simulink model "Lithium0x2DionScaling"  (R2024b)
settings: Solver=FixedStepAuto  StartTime=0.0  StopTime=10  FixedStep=0.001  RelTol=1e-3
libraries: spsControlledCurrentSourceLib x1, spsControlledVoltageSourceLib x1, spsCurrentMeasurementLib x1, spsSeriesRLCBranchLib x1, spsVoltageMeasurementLib x1, spspowerguiLib x1
settings Model: Creator=holthoff  LastModifiedBy=kauchr

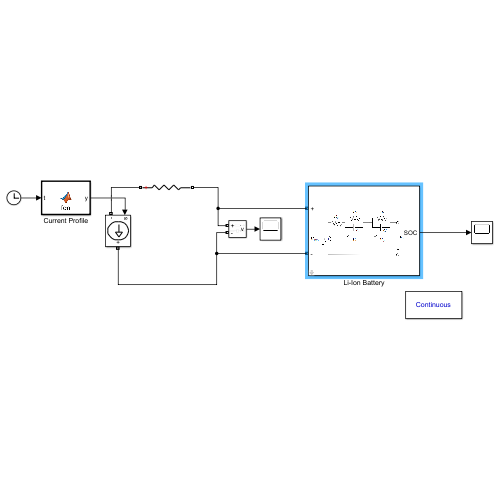
[thumbnail: Simulink's stored preview of the top-level diagram]
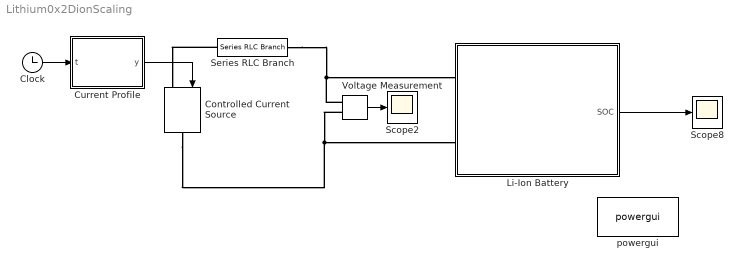
== system Lithium0x2DionScaling ==
  Clock : Clock
  Controlled Current Source : spsControlledCurrentSourceLib/Controlled Current Source  Initialize=off  Source_Type=AC  Amplitude=0  Phase=0  Frequency=0  Measurements=None
  Current Profile : MATLAB Function  TreatAsAtomicUnit=on
  Li-Ion Battery : Subsystem  mask{RCap=2.6, NomV=3.2, soc=50, n=100, m=100}
      mask prompts: RCap "Rated Capacity (Ah)"; NomV "Nominal Voltage (V)"; soc "Initial SOC (%)"; n "Number of cells in series"; m "Number of cells in parallel"
      mask DialogControl DescTextVar Prompt: Lithium-Ion Battery
      mask DialogControl Control2 Prompt: This generic model represents a lithium-ion battery consisting of an arbitrary number of cells connected in series and in parallel. The model is designed to simulate the electrical characteristics of the stack, including current, voltage, and SOC.
      mask Display: image('liion.png', [0,0,20,0,100,100]);
  Scope2 : Scope
  Scope8 : Scope
  Series RLC Branch : spsSeriesRLCBranchLib/Series RLC Branch  LConnTagsString=__new0  RConnTagsString=__new0  BranchType=R  Resistance=1  Inductance=1e-3  SetiL0=off  InitialCurrent=0  Capacitance=1e-6  Setx0=off  InitialVoltage=0  Measurements=None
  Voltage Measurement : spsVoltageMeasurementLib/Voltage Measurement  PhasorSimulation=off  OutputType=Complex  PSBequivalent=0
  powergui : spspowerguiLib/powergui  Priority=1  SimulationMode=Continuous  SampleTime=50e-6  frequency=60  Iterations=50  frequencyindice=0  Pbase=100e6  ErrMax=1e-4  UnitsV=kV  UnitsW=MW  buscounter=0  FunctionMessages=off  echomessages=off  EnableUseOfTLC=off  CurrentSourceSwitches=off  DisableSnubberDevices=off  DisableRonSwitches=off  DisableVfSwitches=off  DisplayEquations=off  AutomaticDiscreteSolvers=off  SolverType=Tustin/Backward Euler (TBE)  Interpol=off  ExternalGateDelay=off  methode=off  Ts=100  x0status=blocks  SPID=on  SwTol=0  HookPort=off  NonlinearTolerance=1e-4  nMaxIteration=100  ContinueOnMaxIteration=off  RestoreLinks=warning  ResistiveCurrentMeasurement=off  Frange=[0:2:500]  Ylog=off  Xlog=on  ShowGrid=off  save=off  variable=ZData  structure=0  ZoomFFT=off  StartTime=0.0  cycles=1  DisplayStyle=1  fundamental=60  FreqAxis=off  MaxFrequency=1000  frequencyindicesteady=1  RmsSteady=1  display=off
  wires:
  Li-Ion Battery/1(SOC) -> Scope8/1
  Clock/1 -> Current Profile/1(t)
  Voltage Measurement/1 -> Scope2/1
  Current Profile/1(y) -> Controlled Current Source/1
  connections:
  Controlled Current Source/RConn1 -- Voltage Measurement/LConn2 -- Li-Ion Battery/LConn2
  Voltage Measurement/LConn1 -- Series RLC Branch/RConn1 -- Li-Ion Battery/LConn1
  Series RLC Branch/LConn1 -- Controlled Current Source/LConn1

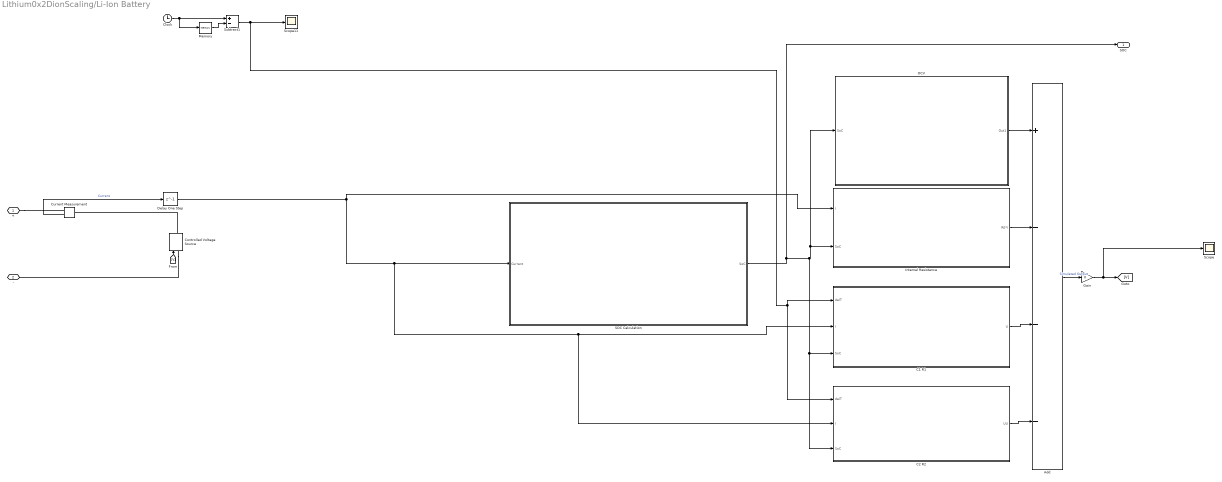
== system Lithium0x2DionScaling/Li-Ion Battery ==
  Add : Sum  Inputs=+---
  C1 R1 : Subsystem
  C2 R2 : Subsystem
  Clock : Clock
  Controlled Voltage Source : spsControlledVoltageSourceLib/Controlled Voltage Source  Initialize=on  Source_Type=AC  Amplitude=0  Phase=0  Frequency=0  Measurements=None
  Current Measurement : spsCurrentMeasurementLib/Current Measurement  PhasorSimulation=off  OutputType=Complex  PSBequivalent=0
  Delay One Step : Delay  DelayLength=1
  Gain : Gain  Gain=n
  Internal Resistance : Subsystem
  Memory : Memory
  OCV : Subsystem
  SOC Calculation : Subsystem
  Scope : Scope
  Scope11 : Scope
  Subtract1 : Sum  Inputs=+-
  + : PMIOPort  Side=Left
  - : PMIOPort  Port=2  Side=Left
  SOC : Outport
  wires:
  Add/1 -> Gain/1  "Simulated Output"
  Clock/1 -> Subtract1/1, Memory/1
  Subtract1/1 -> C2 R2/1(delT), C1 R1/1(delT), Scope11/1
  Memory/1 -> Subtract1/2
  Internal Resistance/1(R0*I) -> Add/2
  OCV/1(Out1) -> Add/1
  C1 R1/1(U) -> Add/3
  C2 R2/1(UU) -> Add/4
  SOC Calculation/1(SoC) -> SOC/1, OCV/1(SoC), Internal Resistance/2(SoC), C2 R2/3(SoC), C1 R1/3(SoC)
  [V] -> Controlled Voltage Source/1
  Current Measurement/1 -> Delay One Step/1  "Current"
  Delay One Step/1 -> C2 R2/2(I), C1 R1/2(I), SOC Calculation/1(Current), Internal Resistance/1(I)
  Gain/1 -> Scope/1, [V]
  connections:
  +/RConn1 -- Current Measurement/RConn1
  Controlled Voltage Source/RConn1 -- Current Measurement/LConn1
  Controlled Voltage Source/LConn1 -- -/RConn1

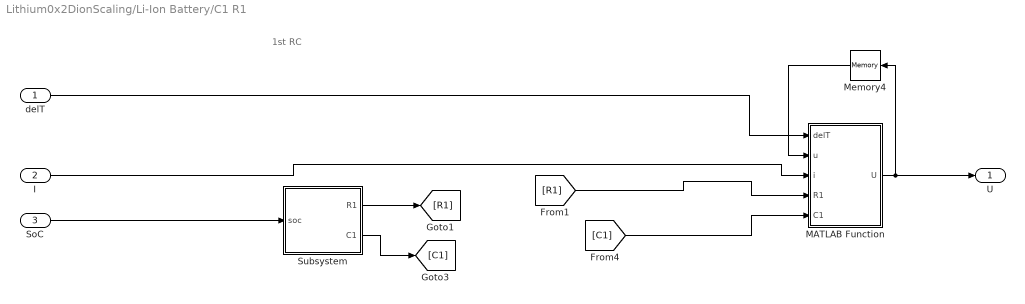
== system Lithium0x2DionScaling/Li-Ion Battery/C1 R1 ==
  note: 1st RC
  delT : Inport
  I : Inport  Port=2
  SoC : Inport  Port=3
  MATLAB Function : MATLAB Function  TreatAsAtomicUnit=on
  Memory4 : Memory
  Subsystem : Subsystem
  U : Outport
  wires:
  Subsystem/1(R1) -> [R1]
  MATLAB Function/1(U) -> U/1, Memory4/1
  delT/1 -> MATLAB Function/1(delT)
  Memory4/1 -> MATLAB Function/2(u)
  [R1] -> MATLAB Function/4(R1)
  Subsystem/2(C1) -> [C1]
  [C1] -> MATLAB Function/5(C1)
  SoC/1 -> Subsystem/1(soc)
  I/1 -> MATLAB Function/3(i)

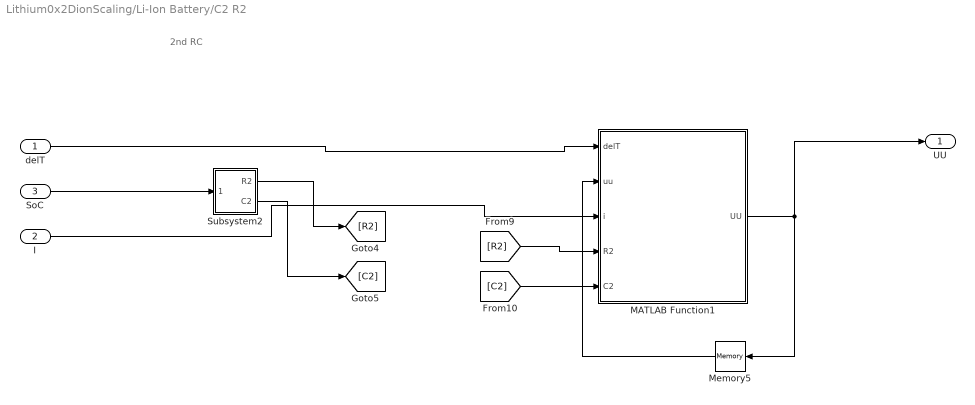
== system Lithium0x2DionScaling/Li-Ion Battery/C2 R2 ==
  note: 2nd RC
  delT : Inport
  I : Inport  Port=2
  SoC : Inport  Port=3
  MATLAB Function1 : MATLAB Function  TreatAsAtomicUnit=on
  Memory5 : Memory
  Subsystem2 : Subsystem
  UU : Outport
  wires:
  [R2] -> MATLAB Function1/4(R2)
  Subsystem2/2(C2) -> [C2]
  Memory5/1 -> MATLAB Function1/2(uu)
  Subsystem2/1(R2) -> [R2]
  [C2] -> MATLAB Function1/5(C2)
  MATLAB Function1/1(UU) -> UU/1, Memory5/1
  SoC/1 -> Subsystem2/1(soc)
  delT/1 -> MATLAB Function1/1(delT)
  I/1 -> MATLAB Function1/3(i)

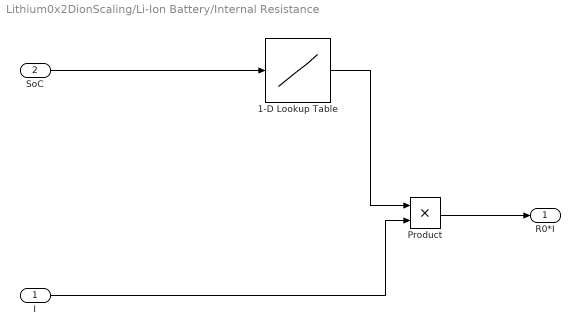
== system Lithium0x2DionScaling/Li-Ion Battery/Internal Resistance ==
  I : Inport
  SoC : Inport  Port=2
  1-D Lookup Table : Lookup_n-D  NumberOfTableDimensions=1  BreakpointsForDimension1=[0;0.01;0.02;0.029999999999999999;0.040000000000000001;0.050000000000000003;0.059999999999999998;0.070000000000000007;0.080000000000000002;0.089999999999999997;0.10000000000000001;0.11;0.12;0.13;0.14000000000000001;0.14999999999999999;0.16;0.17000000000000001;0.17999999999999999;0.19;0.20000000000000001;0.20999999999999999;0.22;0.23000000000000001;0.23999999999999999;0.25;0.26000000000000001;0.27000000000000002;0.28000000000000003;0.28999999999999998;0.29999999999999999;0.31;0.32000000000000001;0.33000000000000002;0.34000000000000002;0.34999999999999998;0.35999999999999999;0.37;0.38;0.39000000000000001;0.40000000000000002;0.40999999999999998;0.41999999999999998;0.42999999999999999;0.44;0.45000000000000001;0.46000000000000002;0.46999999999999997;0.47999999999999998;0.48999999999999999;0.5;0.51000000000000001;0.52000000000000002;0.53000000000000003;0.54000000000000004;0.55000000000000004;0.56000000000000005;0.56999999999999995;0.57999999999999996;0.58999999999999997;0.59999999999999998;0.60999999999999999;0.62;0.63;0.64000000000000001;0.65000000000000002;0.66000000000000003;0.67000000000000004;0.68000000000000005;0.68999999999999995;0.69999999999999996;0.70999999999999996;0.71999999999999997;0.72999999999999998;0.73999999999999999;0.75;0.76000000000000001;0.77000000000000002;0.78000000000000003;0.79000000000000004;0.80000000000000004;0.81000000000000005;0.81999999999999995;0.82999999999999996;0.83999999999999997;0.84999999999999998;0.85999999999999999;0.87;0.88;0.89000000000000001;0.90000000000000002;0.91000000000000003;0.92000000000000004;0.93000000000000005;0.93999999999999995;0.94999999999999996;0.95999999999999996;0.96999999999999997;0.97999999999999998;0.98999999999999999;1]  Table=[0.0263338;0.01843229;0.01552549;0.01445614;0.01406275;0.01391803;0.01386479;0.0138452;0.01383799;0.01383534;0.01383437;0.01383401;0.01383388;0.01383383;0.01383381;0.01383381;0.0138338;0.0138338;0.0138338;0.0138338;0.0138338;0.0138338;0.0138338;0.0138338;0.0138338;0.0138338;0.0138338;0.0138338;0.0138338;0.0138338;0.0138338;0.0138338;0.0138338;0.0138338;0.0138338;0.0138338;0.0138338;0.0138338;0.0138338;0.0138338;0.0138338;0.0138338;0.0138338;0.0138338;0.0138338;0.0138338;0.0138338;0.0138338;0.0138338;0.0138338;0.0138338;0.0138338;0.0138338;0.0138338;0.0138338;0.0138338;0.0138338;0.0138338;0.0138338;0.0138338;0.0138338;0.0138338;0.0138338;0.0138338;0.0138338;0.0138338;0.0138338;0.0138338;0.0138338;0.0138338;0.0138338;0.0138338;0.0138338;0.0138338;0.0138338;0.0138338;0.0138338;0.0138338;0.0138338;0.0138338;0.0138338;0.0138338;0.0138338;0.0138338;0.0138338;0.0138338;0.0138338;0.0138338;0.0138338;0.0138338;0.0138338;0.0138338;0.0138338;0.0138338;0.0138338;0.0138338;0.0138338;0.0138338;0.0138338;0.0138338;0.0138338]  InternalRulePriority=Speed  RndMeth=Simplest
  Product : Product
  R0*I : Outport
  wires:
  Product/1 -> R0*I/1
  SoC/1 -> 1-D Lookup Table/1
  I/1 -> Product/2
  1-D Lookup Table/1 -> Product/1

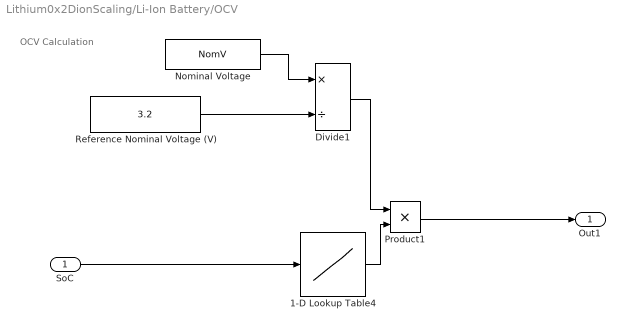
== system Lithium0x2DionScaling/Li-Ion Battery/OCV ==
  note: OCV Calculation
  SoC : Inport
  1-D Lookup Table4 : Lookup_n-D  NumberOfTableDimensions=1  BreakpointsForDimension1=[0;0.01;0.02;0.029999999999999999;0.040000000000000001;0.050000000000000003;0.059999999999999998;0.070000000000000007;0.080000000000000002;0.089999999999999997;0.10000000000000001;0.11;0.12;0.13;0.14000000000000001;0.14999999999999999;0.16;0.17000000000000001;0.17999999999999999;0.19;0.20000000000000001;0.20999999999999999;0.22;0.23000000000000001;0.23999999999999999;0.25;0.26000000000000001;0.27000000000000002;0.28000000000000003;0.28999999999999998;0.29999999999999999;0.31;0.32000000000000001;0.33000000000000002;0.34000000000000002;0.34999999999999998;0.35999999999999999;0.37;0.38;0.39000000000000001;0.40000000000000002;0.40999999999999998;0.41999999999999998;0.42999999999999999;0.44;0.45000000000000001;0.46000000000000002;0.46999999999999997;0.47999999999999998;0.48999999999999999;0.5;0.51000000000000001;0.52000000000000002;0.53000000000000003;0.54000000000000004;0.55000000000000004;0.56000000000000005;0.56999999999999995;0.57999999999999996;0.58999999999999997;0.59999999999999998;0.60999999999999999;0.62;0.63;0.64000000000000001;0.65000000000000002;0.66000000000000003;0.67000000000000004;0.68000000000000005;0.68999999999999995;0.69999999999999996;0.70999999999999996;0.71999999999999997;0.72999999999999998;0.73999999999999999;0.75;0.76000000000000001;0.77000000000000002;0.78000000000000003;0.79000000000000004;0.80000000000000004;0.81000000000000005;0.81999999999999995;0.82999999999999996;0.83999999999999997;0.84999999999999998;0.85999999999999999;0.87;0.88;0.89000000000000001;0.90000000000000002;0.91000000000000003;0.92000000000000004;0.93000000000000005;0.93999999999999995;0.94999999999999996;0.95999999999999996;0.96999999999999997;0.97999999999999998;0.98999999999999999;1]  Table=[3.29571729606682;3.32213631956766;3.34664360147367;3.36934563044947;3.39034548891849;3.40974290407478;3.42763429889471;3.44411284314879;3.45926850441342;3.47318809908262;3.48595534337984;3.49765090436971;3.50835245096978;3.51813470496231;3.52706949200605;3.53522579264794;3.54266979333496;3.54946493742581;3.55567197620274;3.56134901988328;3.56655158863201;3.57133266357232;3.5757427377982;3.57982986738595;3.58363972240603;3.58721563793471;3.59059866506595;3.59382762192308;3.59693914467061;3.59996773852596;3.60294582877126;3.60590381176509;3.60887010595426;3.61187120288554;3.61493171821749;3.61807444273214;3.62132039334682;3.62468886412591;3.62819747729257;3.63186223424055;3.63569756654593;3.63971638697887;3.64393014051541;3.64834885534923;3.65298119390336;3.65783450384201;3.66291486908231;3.66822716080606;3.67377508847152;3.67956125082515;3.68558718691339;3.69185342709441;3.69835954404988;3.70510420379676;3.71208521669903;3.71929958847944;3.72674357123133;3.73441271443036;3.74230191594627;3.75040547305464;3.75871713344867;3.76723014625097;3.77593731302525;3.78483103878816;3.793903383021;3.80314611068152;3.81255074321565;3.82210860956932;3.83181089720015;3.84164870308928;3.85161308475308;3.86169511125496;3.87188591421712;3.88217673883228;3.8925589948755;3.90302430771591;3.91356456932847;3.92417198930575;3.9348391458697;3.94555903688339;3.95632513086279;3.96713141798853;3.97797246111767;3.98884344679546;3.99974023626709;4.01065941648949;4.02159835114304;4.03255523164341;4.04352912815324;4.05452004059395;4.06552894965752;4.07655786781822;4.08760989034436;4.09868924631014;4.10980134960729;4.12095284995694;4.13215168392133;4.14340712591558;4.15472983921947;4.16613192698919;4.17762698326911]  InternalRulePriority=Speed  RndMeth=Simplest
  Divide1 : Product  Inputs=*/
  Nominal Voltage : Constant  Value=NomV
  Product1 : Product
  Reference Nominal Voltage (V) : Constant  Value=3.2
  Out1 : Outport
  wires:
  Product1/1 -> Out1/1
  1-D Lookup Table4/1 -> Product1/2
  SoC/1 -> 1-D Lookup Table4/1
  Reference Nominal Voltage (V)/1 -> Divide1/2
  Divide1/1 -> Product1/1
  Nominal Voltage/1 -> Divide1/1

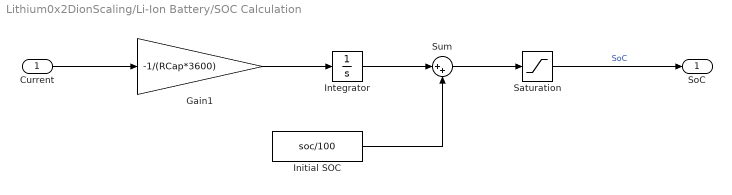
== system Lithium0x2DionScaling/Li-Ion Battery/SOC Calculation ==
  Current : Inport
  Gain1 : Gain  Gain=-1/(RCap*3600)
  Initial SOC : Constant  Value=soc/100
  Integrator : Integrator
  Saturation : Saturate  UpperLimit=1  LowerLimit=0
  Sum : Sum  Inputs=|++
  SoC : Outport
  wires:
  Current/1 -> Gain1/1
  Gain1/1 -> Integrator/1
  Integrator/1 -> Sum/1
  Initial SOC/1 -> Sum/2
  Sum/1 -> Saturation/1
  Saturation/1 -> SoC/1  "SoC"

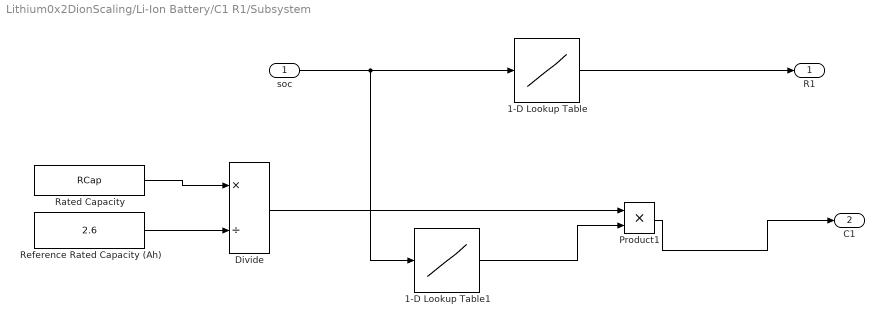
== system Lithium0x2DionScaling/Li-Ion Battery/C1 R1/Subsystem ==
  soc : Inport
  " Rated Capacity" : Constant  Value=RCap
  1-D Lookup Table : Lookup_n-D  NumberOfTableDimensions=1  BreakpointsForDimension1=[0;0.01;0.02;0.029999999999999999;0.040000000000000001;0.050000000000000003;0.059999999999999998;0.070000000000000007;0.080000000000000002;0.089999999999999997;0.10000000000000001;0.11;0.12;0.13;0.14000000000000001;0.14999999999999999;0.16;0.17000000000000001;0.17999999999999999;0.19;0.20000000000000001;0.20999999999999999;0.22;0.23000000000000001;0.23999999999999999;0.25;0.26000000000000001;0.27000000000000002;0.28000000000000003;0.28999999999999998;0.29999999999999999;0.31;0.32000000000000001;0.33000000000000002;0.34000000000000002;0.34999999999999998;0.35999999999999999;0.37;0.38;0.39000000000000001;0.40000000000000002;0.40999999999999998;0.41999999999999998;0.42999999999999999;0.44;0.45000000000000001;0.46000000000000002;0.46999999999999997;0.47999999999999998;0.48999999999999999;0.5;0.51000000000000001;0.52000000000000002;0.53000000000000003;0.54000000000000004;0.55000000000000004;0.56000000000000005;0.56999999999999995;0.57999999999999996;0.58999999999999997;0.59999999999999998;0.60999999999999999;0.62;0.63;0.64000000000000001;0.65000000000000002;0.66000000000000003;0.67000000000000004;0.68000000000000005;0.68999999999999995;0.69999999999999996;0.70999999999999996;0.71999999999999997;0.72999999999999998;0.73999999999999999;0.75;0.76000000000000001;0.77000000000000002;0.78000000000000003;0.79000000000000004;0.80000000000000004;0.81000000000000005;0.81999999999999995;0.82999999999999996;0.83999999999999997;0.84999999999999998;0.85999999999999999;0.87;0.88;0.89000000000000001;0.90000000000000002;0.91000000000000003;0.92000000000000004;0.93000000000000005;0.93999999999999995;0.94999999999999996;0.95999999999999996;0.96999999999999997;0.97999999999999998;0.98999999999999999;1]  Table=[0.025;0.01709849;0.01419169;0.01312234;0.01272895;0.01258422;0.01253098;0.0125114;0.01250419;0.01250154;0.01250057;0.01250021;0.01250008;0.01250003;0.01250001;0.0125;0.0125;0.0125;0.0125;0.0125;0.0125;0.0125;0.0125;0.0125;0.0125;0.0125;0.0125;0.0125;0.0125;0.0125;0.0125;0.0125;0.0125;0.0125;0.0125;0.0125;0.0125;0.0125;0.0125;0.0125;0.0125;0.0125;0.0125;0.0125;0.0125;0.0125;0.0125;0.0125;0.0125;0.0125;0.0125;0.0125;0.0125;0.0125;0.0125;0.0125;0.0125;0.0125;0.0125;0.0125;0.0125;0.0125;0.0125;0.0125;0.0125;0.0125;0.0125;0.0125;0.0125;0.0125;0.0125;0.0125;0.0125;0.0125;0.0125;0.0125;0.0125;0.0125;0.0125;0.0125;0.0125;0.0125;0.0125;0.0125;0.0125;0.0125;0.0125;0.0125;0.0125;0.0125;0.0125;0.0125;0.0125;0.0125;0.0125;0.0125;0.0125;0.0125;0.0125;0.0125;0.0125]  InternalRulePriority=Speed  RndMeth=Simplest
  1-D Lookup Table1 : Lookup_n-D  NumberOfTableDimensions=1  BreakpointsForDimension1=[0;0.01;0.02;0.029999999999999999;0.040000000000000001;0.050000000000000003;0.059999999999999998;0.070000000000000007;0.080000000000000002;0.089999999999999997;0.10000000000000001;0.11;0.12;0.13;0.14000000000000001;0.14999999999999999;0.16;0.17000000000000001;0.17999999999999999;0.19;0.20000000000000001;0.20999999999999999;0.22;0.23000000000000001;0.23999999999999999;0.25;0.26000000000000001;0.27000000000000002;0.28000000000000003;0.28999999999999998;0.29999999999999999;0.31;0.32000000000000001;0.33000000000000002;0.34000000000000002;0.34999999999999998;0.35999999999999999;0.37;0.38;0.39000000000000001;0.40000000000000002;0.40999999999999998;0.41999999999999998;0.42999999999999999;0.44;0.45000000000000001;0.46000000000000002;0.46999999999999997;0.47999999999999998;0.48999999999999999;0.5;0.51000000000000001;0.52000000000000002;0.53000000000000003;0.54000000000000004;0.55000000000000004;0.56000000000000005;0.56999999999999995;0.57999999999999996;0.58999999999999997;0.59999999999999998;0.60999999999999999;0.62;0.63;0.64000000000000001;0.65000000000000002;0.66000000000000003;0.67000000000000004;0.68000000000000005;0.68999999999999995;0.69999999999999996;0.70999999999999996;0.71999999999999997;0.72999999999999998;0.73999999999999999;0.75;0.76000000000000001;0.77000000000000002;0.78000000000000003;0.79000000000000004;0.80000000000000004;0.81000000000000005;0.81999999999999995;0.82999999999999996;0.83999999999999997;0.84999999999999998;0.85999999999999999;0.87;0.88;0.89000000000000001;0.90000000000000002;0.91000000000000003;0.92000000000000004;0.93000000000000005;0.93999999999999995;0.94999999999999996;0.95999999999999996;0.96999999999999997;0.97999999999999998;0.98999999999999999;1]  Table=[49;49.3934693402873;49.6321205588285;49.7768698398515;49.8646647167634;49.9179150013761;49.9502129316321;49.9698026165777;49.9816843611112;49.9888910034617;49.9932620530009;49.9959132285615;49.9975212478233;49.998496560807;49.9990881180344;49.9994469156298;49.9996645373721;49.999796531631;49.9998765901959;49.9999251481701;49.9999546000702;49.9999724635506;49.9999832982992;49.9999898699064;49.9999938557876;49.9999962733468;49.9999977396706;49.9999986290409;49.9999991684713;49.9999994956523;49.9999996940977;49.9999998144608;49.9999998874648;49.9999999317439;49.9999999586006;49.99999997489;49.99999998477;49.9999999907625;49.9999999943972;49.9999999966017;49.9999999979388;49.9999999987498;49.9999999992417;49.9999999995401;49.999999999721;49.9999999998308;49.9999999998974;49.9999999999377;49.9999999999622;49.9999999999771;49.9999999999861;49.9999999999916;49.9999999999949;49.9999999999969;49.9999999999981;49.9999999999988;49.9999999999993;49.9999999999996;49.9999999999997;49.9999999999998;49.9999999999999;49.9999999999999;49.9999999999999;50;50;50;50;50;50;50;50;50;50;50;50;50;50;50;50;50;50;50;50;50;50;50;50;50;50;50;50;50;50;50;50;50;50;50;50;50;50]  InternalRulePriority=Speed  RndMeth=Simplest
  Divide : Product  Inputs=*/
  Product1 : Product
  Reference Rated Capacity (Ah) : Constant  Value=2.6
  R1 : Outport
  C1 : Outport  Port=2
  wires:
  soc/1 -> 1-D Lookup Table1/1, 1-D Lookup Table/1
  1-D Lookup Table1/1 -> Product1/2
  Reference Rated Capacity (Ah)/1 -> Divide/2
  Divide/1 -> Product1/1
  " Rated Capacity"/1 -> Divide/1
  Product1/1 -> C1/1
  1-D Lookup Table/1 -> R1/1

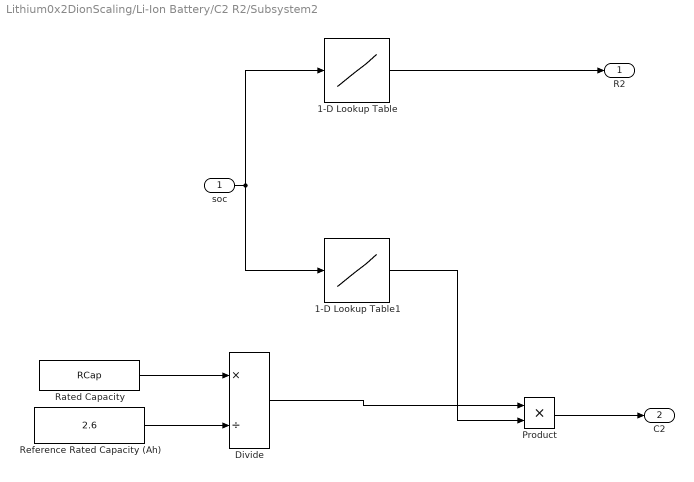
== system Lithium0x2DionScaling/Li-Ion Battery/C2 R2/Subsystem2 ==
  soc : Inport
  " Rated Capacity" : Constant  Value=RCap
  1-D Lookup Table : Lookup_n-D  NumberOfTableDimensions=1  BreakpointsForDimension1=[0;0.01;0.02;0.029999999999999999;0.040000000000000001;0.050000000000000003;0.059999999999999998;0.070000000000000007;0.080000000000000002;0.089999999999999997;0.10000000000000001;0.11;0.12;0.13;0.14000000000000001;0.14999999999999999;0.16;0.17000000000000001;0.17999999999999999;0.19;0.20000000000000001;0.20999999999999999;0.22;0.23000000000000001;0.23999999999999999;0.25;0.26000000000000001;0.27000000000000002;0.28000000000000003;0.28999999999999998;0.29999999999999999;0.31;0.32000000000000001;0.33000000000000002;0.34000000000000002;0.34999999999999998;0.35999999999999999;0.37;0.38;0.39000000000000001;0.40000000000000002;0.40999999999999998;0.41999999999999998;0.42999999999999999;0.44;0.45000000000000001;0.46000000000000002;0.46999999999999997;0.47999999999999998;0.48999999999999999;0.5;0.51000000000000001;0.52000000000000002;0.53000000000000003;0.54000000000000004;0.55000000000000004;0.56000000000000005;0.56999999999999995;0.57999999999999996;0.58999999999999997;0.59999999999999998;0.60999999999999999;0.62;0.63;0.64000000000000001;0.65000000000000002;0.66000000000000003;0.67000000000000004;0.68000000000000005;0.68999999999999995;0.69999999999999996;0.70999999999999996;0.71999999999999997;0.72999999999999998;0.73999999999999999;0.75;0.76000000000000001;0.77000000000000002;0.78000000000000003;0.79000000000000004;0.80000000000000004;0.81000000000000005;0.81999999999999995;0.82999999999999996;0.83999999999999997;0.84999999999999998;0.85999999999999999;0.87;0.88;0.89000000000000001;0.90000000000000002;0.91000000000000003;0.92000000000000004;0.93000000000000005;0.93999999999999995;0.94999999999999996;0.95999999999999996;0.96999999999999997;0.97999999999999998;0.98999999999999999;1]  Table=[0.025;0.01419169;0.01272895;0.01253098;0.01250419;0.01250057;0.01250008;0.01250001;0.0125;0.0125;0.0125;0.0125;0.0125;0.0125;0.0125;0.0125;0.0125;0.0125;0.0125;0.0125;0.0125;0.0125;0.0125;0.0125;0.0125;0.0125;0.0125;0.0125;0.0125;0.0125;0.0125;0.0125;0.0125;0.0125;0.0125;0.0125;0.0125;0.0125;0.0125;0.0125;0.0125;0.0125;0.0125;0.0125;0.0125;0.0125;0.0125;0.0125;0.0125;0.0125;0.0125;0.0125;0.0125;0.0125;0.0125;0.0125;0.0125;0.0125;0.0125;0.0125;0.0125;0.0125;0.0125;0.0125;0.0125;0.0125;0.0125;0.0125;0.0125;0.0125;0.0125;0.0125;0.0125;0.0125;0.0125;0.0125;0.0125;0.0125;0.0125;0.0125;0.0125;0.0125;0.0125;0.0125;0.0125;0.0125;0.0125;0.0125;0.0125;0.0125;0.0125;0.0125;0.0125;0.0125;0.0125;0.0125;0.0125;0.0125;0.0125;0.0125;0.0125]  InternalRulePriority=Speed  RndMeth=Simplest
  1-D Lookup Table1 : Lookup_n-D  NumberOfTableDimensions=1  BreakpointsForDimension1=[0;0.01;0.02;0.029999999999999999;0.040000000000000001;0.050000000000000003;0.059999999999999998;0.070000000000000007;0.080000000000000002;0.089999999999999997;0.10000000000000001;0.11;0.12;0.13;0.14000000000000001;0.14999999999999999;0.16;0.17000000000000001;0.17999999999999999;0.19;0.20000000000000001;0.20999999999999999;0.22;0.23000000000000001;0.23999999999999999;0.25;0.26000000000000001;0.27000000000000002;0.28000000000000003;0.28999999999999998;0.29999999999999999;0.31;0.32000000000000001;0.33000000000000002;0.34000000000000002;0.34999999999999998;0.35999999999999999;0.37;0.38;0.39000000000000001;0.40000000000000002;0.40999999999999998;0.41999999999999998;0.42999999999999999;0.44;0.45000000000000001;0.46000000000000002;0.46999999999999997;0.47999999999999998;0.48999999999999999;0.5;0.51000000000000001;0.52000000000000002;0.53000000000000003;0.54000000000000004;0.55000000000000004;0.56000000000000005;0.56999999999999995;0.57999999999999996;0.58999999999999997;0.59999999999999998;0.60999999999999999;0.62;0.63;0.64000000000000001;0.65000000000000002;0.66000000000000003;0.67000000000000004;0.68000000000000005;0.68999999999999995;0.69999999999999996;0.70999999999999996;0.71999999999999997;0.72999999999999998;0.73999999999999999;0.75;0.76000000000000001;0.77000000000000002;0.78000000000000003;0.79000000000000004;0.80000000000000004;0.81000000000000005;0.81999999999999995;0.82999999999999996;0.83999999999999997;0.84999999999999998;0.85999999999999999;0.87;0.88;0.89000000000000001;0.90000000000000002;0.91000000000000003;0.92000000000000004;0.93000000000000005;0.93999999999999995;0.94999999999999996;0.95999999999999996;0.96999999999999997;0.97999999999999998;0.98999999999999999;1]  Table=[299;299.632120558828;299.864664716763;299.950212931632;299.981684361111;299.993262053001;299.997521247823;299.999088118034;299.999664537372;299.999876590196;299.99995460007;299.999983298299;299.999993855787;299.99999773967;299.999999168471;299.999999694097;299.999999887464;299.9999999586;299.99999998477;299.999999994397;299.999999997939;299.999999999241;299.999999999721;299.999999999897;299.999999999962;299.999999999986;299.999999999995;299.999999999998;299.999999999999;299.999999999999;300;300;300;300;300;300;300;300;300;300;300;300;300;300;300;300;300;300;300;300;300;300;300;300;300;300;300;300;300;300;300;300;300;300;300;300;300;300;300;300;300;300;300;300;300;300;300;300;300;300;300;300;300;300;300;300;300;300;300;300;300;300;300;300;300;300;300;300;300;300;300]  InternalRulePriority=Speed  RndMeth=Simplest
  Divide : Product  Inputs=*/
  Product : Product
  Reference Rated Capacity (Ah) : Constant  Value=2.6
  R2 : Outport
  C2 : Outport  Port=2
  wires:
  1-D Lookup Table1/1 -> Product/2
  soc/1 -> 1-D Lookup Table1/1, 1-D Lookup Table/1
  Divide/1 -> Product/1
  Reference Rated Capacity (Ah)/1 -> Divide/2
  " Rated Capacity"/1 -> Divide/1
  Product/1 -> C2/1
  1-D Lookup Table/1 -> R2/1

== matlab function Lithium0x2DionScaling/Li-Ion Battery/C1 R1/MATLAB Function ==
  data: delT input; U output; u input; i input; R1 input; C1 input
function U    = fcn(delT,u, i, R1,C1)


 U = (exp(-delT/(R1*C1))*u)+(R1*(1-exp(-delT/(R1*C1)))*i);

== matlab function Lithium0x2DionScaling/Li-Ion Battery/C2 R2/MATLAB Function1 ==
  data: delT input; UU output; uu input; i input; R2 input; C2 input
function UU    = fcn(delT,uu, i, R2,C2)


 UU = (exp(-delT/(R2*C2))*uu)+(R2*(1-exp(-delT/(R2*C2)))*i);

== matlab function Lithium0x2DionScaling/Current Profile ==
  data: t input; y output
function y = fcn(t)
    ts = 0.001; % s
    t0 = 0;     % s
    tend = 5;   % s

    if t < t0 || t > tend
        y = 0; 
        return;
    end

    ms1 = 1.99; % s
    ms2 = 2;
    ms3 = 3;
    ms4 = 3.01;

    interval1 = t >= t0 && t < ms1;
    interval2 = t >= ms1 && t < ms2;
    interval3 = t >= ms2 && t < ms3;
    interval4 = t >= ms3 && t < ms4;
    interval5 = t >= ms4 && t <= tend;

    fvseg1 = 0;     % Final value of interval
    fvseg2 = 30;  % Rated maximum current peak current for 1 s in A
    fvseg3 = 30;
    fvseg4 = -32.5;
    fvseg5 = -32.5;

    if interval1
        y = fvseg1; 
    elseif interval2
        % Ramp up
        y = fvseg1 + (fvseg2 - fvseg1) * ((t - ms1) / (ms2 - ms1));
    elseif interval3
        y = fvseg3; 
    elseif interval4
        % Ramp down
        y = fvseg3 + (fvseg4 - fvseg3) * ((t - ms3) / (ms4 - ms3));
    else
        y = fvseg5;
    end
end
